simulink model "MEX_MDL_UDP_test"  (R2022b)
settings: Solver=VariableStepAuto  StartTime=0.0  StopTime=10.0  RelTol=1e-3
libraries: slrealtimeutilitieslib x2, sldrtlib x1
settings Model: Creator=javnson  LastModifiedBy=javnson

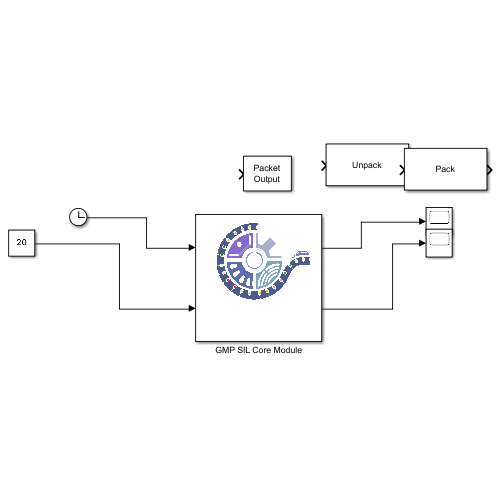
[thumbnail: Simulink's stored preview of the top-level diagram]
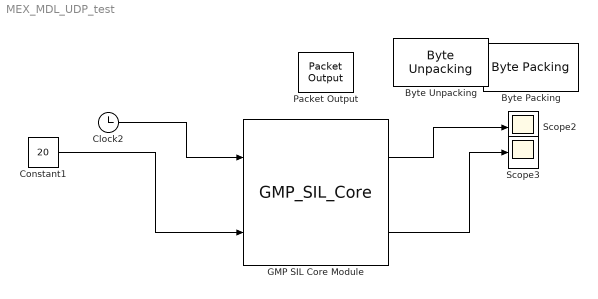
== system MEX_MDL_UDP_test ==
  Byte Packing : slrealtimeutilitieslib/Byte Packing  MaskPackedDataType=uint8  MaskUnpackedDataTypes={'uint8'}  MaskAlignment=1
  Byte Unpacking : slrealtimeutilitieslib/Byte Unpacking  MaskUnpackedDataTypes={'uint8'}  MaskUnpackedDataSizes={[1]}  MaskAlignment=1
  Clock2 : Clock
  Constant1 : Constant  Value=20
  GMP SIL Core Module : S-Function  FunctionName=GMP_SIL_Core  Parameters=NumberUnpackedPorts, UnpackedDataTypes, UnpackedDataSizes, NumberPackedPorts, PackedDataTypes, PackedDataSizes, Alignment, HostAddr, TargetPort  SFunctionDeploymentMode=off  EnableBusSupport=off  mask{MaskPackedDataTypes={'double','double'}, MaskPackedDataSizes={[1],[1]}, MaskUnpackedDataTypes={'double','double'}, MaskUnpackedDataSizes={[1],[1]}, MaskAlignment=1, MaskHostAddr='127.0.0.1', MaskMsgTxPort=12300, MaskMsgRxPort=12301, MaskCmdTxPort=12302, MaskCmdRxPort=12303}
      mask init:
      | % MDL invoke parameters
      | % NumberUnpackedPorts, UnpackedDataTypes, UnpackedDataSizes, 
      | % NumberPackedPorts, PackedDataTypes, PackedDataSizes, 
      | % Alignment
      | 
      | % source: MaskUnpackedDataTypes, MaskUnpackedDataSizes
      | % source: MaskPackedDataTypes, MaskUnpackedDataSizes
      | % source: MaskAlignment
      | [NumberUnpackedPorts, UnpackedDataTypes, UnpackedDataSizes, ...
      |      NumberPackedPorts, PackedDataTypes, PackedDataSizes, ...
      |      Alignment] = mdl_gmp_simulink_core( ...
      |      MaskUnpackedDataTypes, MaskUnpackedDataSizes, ...
      |      MaskPackedDataTypes, MaskPackedDataSizes,...
      |      MaskAlignment);
      | 
      | % source: MaskHostAddr
      | % source: MaskMsgTxPort, MaskMsgRxPort
      | % source: MaskCmdTxPort, MaskCmdRxPort
      | [HostAddr, TargetPort] = mdl_gmp_simulink_connection(MaskHostAddr, ...
      | 	MaskMsgTxPort, MaskMsgRxPort, ... 
      | 	MaskCmdTxPort, MaskCmdRxPort);
      mask TypeOptions MaskAlignment: 1 | 2 | 4 | 8
      mask DialogControl ParameterGroupVar Prompt: Parameters:
      mask DialogControl Container5 Prompt: Message
      mask DialogControl Control3 Prompt: Data (sent) types (cell array):(pack)
      mask DialogControl Control7 Prompt: Data (send) port dimisions (cell array) (pack), disabled
      mask DialogControl Control5 Prompt: Data (received) types (cell array):(unpack)
      mask DialogControl Control6 Prompt: Data (received) port dimisions (cell array)(unpacked)
      mask DialogControl Control4 Prompt: Byte Alignment:
      mask DialogControl Container6 Prompt: Connection
      mask DialogControl Control8 Prompt: Target Host:
      mask DialogControl Control9 Prompt: MSG Transmit Port:
      mask DialogControl Control10 Prompt: MSG Receive Port:
      mask DialogControl Container7 Prompt: Command Ports
      mask DialogControl Control11 Prompt: CMD Transmit Port:
      mask DialogControl Control12 Prompt: CMD Receive Port:
      mask Display:
      | image('E:\lib\gmp_pro\ctl\simulink_lib\simulink_lib_src\icon\GMP_Core.png');
      | 
      | text(0.5, 0.5, 'GMP SIL CORE Module', horizontalAlignment = 'center',verticalAlignment = 'base');
  Packet Output : sldrtlib/Packet Output  SampleTime=0.1  MaxMissedTicks=10  ShowMissedTicks=off  YieldWhenWaiting=off  DrvAddress=0  DrvOptions=0  PacketSize=32  DataTypes='4*double'  ShowReady=off  ShowError=off  PacketID=1  ByteOrder=1  InitialValue=[]  FinalValue=[]
  Scope2 : Scope
  Scope3 : Scope
  wires:
  GMP SIL Core Module/2 -> Scope3/1
  GMP SIL Core Module/1 -> Scope2/1
  Clock2/1 -> GMP SIL Core Module/1
  Constant1/1 -> GMP SIL Core Module/2
